simulink model "my_model"  (R2024b)
settings: Solver=FixedStepAuto  StartTime=0.0  StopTime=10.0  RelTol=1e-3
undefined symbols (not defined in the file or in its folder): net
libraries: dlconvfclib x3, dlactivationlib x2
settings Model: Creator=xpess  LastModifiedBy=xpess
settings OptimizationCC: DefaultParameterBehavior=Inlined  EnhancedBackFolding=on  PassReuseOutputArgsAs=Individual arguments  ZeroExternalMemoryAtStartup=off  ZeroInternalMemoryAtStartup=off  OptimizeBlockOrder=speed  DifferentSizesBufferReuse=on  OptimizationCustomize=off  EfficientTunableParamExpr=on
settings DebuggingCC: ParameterTunabilityLossMsg=error
settings SFSimCC: MATLABDynamicMemAlloc=off
settings RTWCC: Description=Embedded Coder  SystemTargetFile=ert.tlc  TemplateMakefile=ert_default_tmf
settings CodeAppCC: ForceParamTrailComments=on  IgnoreCustomStorageClasses=off  OperatorAnnotations=on  SimulinkDataObjDesc=on  SFDataObjDesc=on  InsertBlockDesc=on
settings ERTTargetCC: TargetLangStandard=C99 (ISO)  GenerateSampleERTMain=on  ERTCustomFileTemplate=example_file_process.tlc

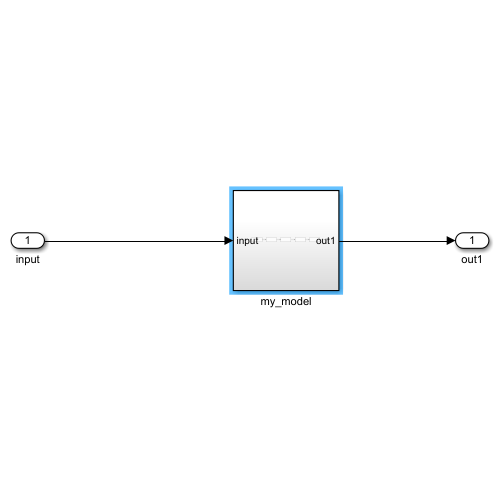
[thumbnail: Simulink's stored preview of the top-level diagram]
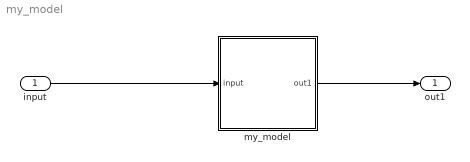
== system my_model ==
  input : Inport  PortDimensions=[4]
  my_model : Subsystem
  out1 : Outport
  wires:
  input/1 -> my_model/1(input)
  my_model/1(out1) -> out1/1

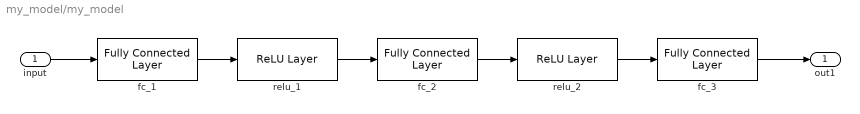
== system my_model/my_model ==
  input : Inport  PortDimensions=[4]
  fc_1 : dlconvfclib/Fully Connected Layer  Layer=net.Layers(2)  OutMin=[]  OutMax=[]  WeightsDataTypeStr=Inherit: Inherit via back propagation  WeightsMin=[]  WeightsMax=[]  BiasDataTypeStr=Inherit: Inherit via back propagation  BiasMin=[]  BiasMax=[]  MatrixMultiplyMin=[]  MatrixMultiplyMax=[]  SampleTime=-1
      settings: DataFormat=C
  fc_2 : dlconvfclib/Fully Connected Layer  Layer=net.Layers(4)  OutMin=[]  OutMax=[]  WeightsDataTypeStr=Inherit: Inherit via back propagation  WeightsMin=[]  WeightsMax=[]  BiasDataTypeStr=Inherit: Inherit via back propagation  BiasMin=[]  BiasMax=[]  MatrixMultiplyMin=[]  MatrixMultiplyMax=[]  SampleTime=-1
      settings: DataFormat=C
  fc_3 : dlconvfclib/Fully Connected Layer  Layer=net.Layers(6)  OutMin=[]  OutMax=[]  WeightsDataTypeStr=Inherit: Inherit via back propagation  WeightsMin=[]  WeightsMax=[]  BiasDataTypeStr=Inherit: Inherit via back propagation  BiasMin=[]  BiasMax=[]  MatrixMultiplyMin=[]  MatrixMultiplyMax=[]  SampleTime=-1
      settings: DataFormat=C
  relu_1 : dlactivationlib/ReLU Layer  OutMin=[]  OutMax=[]  SampleTime=-1
  relu_2 : dlactivationlib/ReLU Layer  OutMin=[]  OutMax=[]  SampleTime=-1
  out1 : Outport
  wires:
  relu_1/1 -> fc_2/1
  fc_3/1 -> out1/1
  input/1 -> fc_1/1
  relu_2/1 -> fc_3/1
  fc_1/1 -> relu_1/1
  fc_2/1 -> relu_2/1
